simulink library "LIB_TF_G_12_StepControl"  (Simulink 8.6)
settings: Solver=ode45  StartTime=0.0  StopTime=10.0  RelTol=1e-3
PreLoadFcn:
  | if exist('tl_preloadfcn','file'), tl_preloadfcn(gcs,402); end
PostLoadFcn:
  | if exist('tl_postloadfcn','file'), tl_postloadfcn(gcs,402); end
undefined symbols (not defined in the file): ddv, u2, u3
libraries: tllib x4, LIB_TF_G_12_StepControl x1
(part 2 of 7)

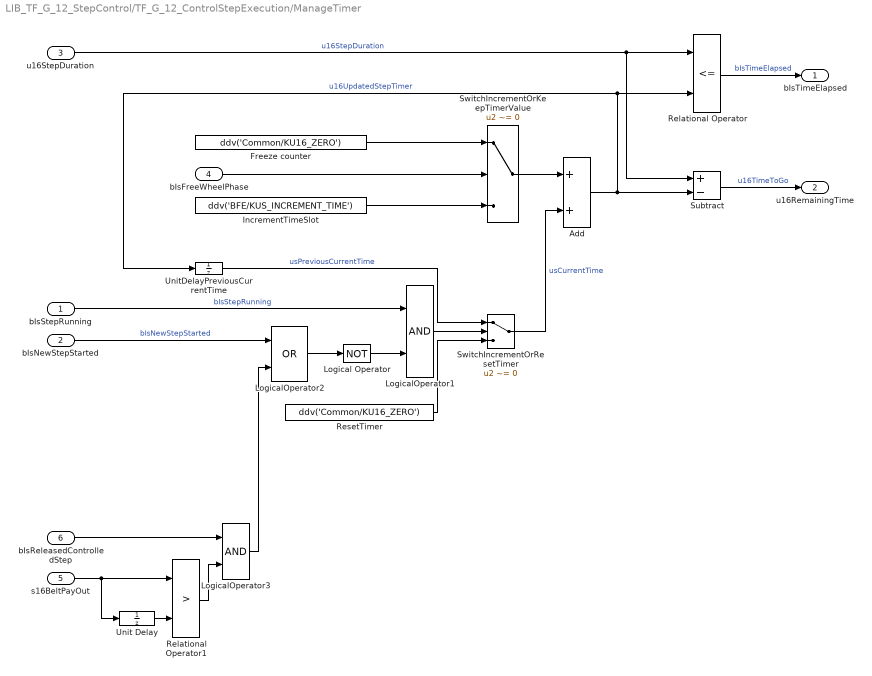
== system LIB_TF_G_12_StepControl/TF_G_12_ControlStepExecution/ManageTimer ==
  bIsStepRunning : Inport  RequirementInfo={} %GIDa_8099bea4_e8c1_4692_a6f9_d176147f505d
  bIsNewStepStarted : Inport  RequirementInfo={} %GIDa_5064309f_314f_43a7_8546_a3acea29a31d  Port=2
  u16StepDuration : Inport  RequirementInfo={} %GIDa_e2682689_4f53_4bd0_88ce_17de940b29c4  Port=3
  bIsFreeWheelPhase : Inport  RequirementInfo={} %GIDa_001aab12_c4fd_412a_b4f3_496d187da0da  Port=4
  s16BeltPayOut : Inport  RequirementInfo={} %GIDa_5cd29b0f_0f87_4eb9_b600_93c60318ecd2  Port=5  OutDataTypeStr=int16
  bIsReleasedControlledStep : Inport  RequirementInfo={} %GIDa_931de2e6_9d0e_47b7_b3af_677f90c0aa82  Port=6
  Add : Sum  RequirementInfo={} %GIDa_29793857_171b_4407_b062_784dd89fa0d8  OutDataTypeStr=uint16  SaturateOnIntegerOverflow=on  mask(TL_Sum){data={'output',{'name','u16UpdatedStepTimer','type','UInt16','checkmin',1,'checkmax',1},'autoscaling',{'mode',2},'date',735951.66800328705}}
      settings: AttributesFormatString=Saturation: %<SaturateOnIntegerOverflow>  CopyFcn=if exist('tl_reset_reviewflag','file')==2,tl_reset_reviewflag(gcbh);end  DeleteFcn=if exist('delete_tlblock','file')==2,delete_tlblock(gcbh);end  NameChangeFcn=if exist('rename_tlblock','file')==2,rename_tlblock(gcbh);end  OpenFcn=if exist('tl_open_blockdlg','file')==2,tl_open_blockdlg(gcbh);else,open_system(gcbh,'parameter');end
      mask Help: eval(['if exist(''tl_online_help'',''file'') == 2, tl_online_help(''Topic'',''TL_Sum''),else, web([''jar:file:///'',matlabroot,''/help/toolbox/simulink/help.jar!/slref/' lower(get_param(gcbh,'Blocktype')) '.html''], ''-helpbrowser''),end'])
      mask Display: plot([-0.05, 1.05, NaN, -0.05, 1.05],[.01, .01, NaN, .99, .99])
  Freeze counter : Constant  RequirementInfo={} %GIDa_b2dcc360_8c19_4b3e_bcea_e2e7e3051644  Value=ddv('Common/KU16_ZERO')  OutDataTypeStr=uint16  mask(TL_Constant){data={'output',{'variable','Common/KU16_ZERO'},'date',735951.66800163197}}
      settings: CopyFcn=if exist('tl_reset_reviewflag','file')==2,tl_reset_reviewflag(gcbh);end  DeleteFcn=if exist('delete_tlblock','file')==2,delete_tlblock(gcbh);end  NameChangeFcn=if exist('rename_tlblock','file')==2,rename_tlblock(gcbh);end  OpenFcn=if exist('tl_open_blockdlg','file')==2,tl_open_blockdlg(gcbh);else,open_system(gcbh,'parameter');end
      mask Help: eval(['if exist(''tl_online_help'',''file'') == 2, tl_online_help(''Topic'',''TL_Constant''),else, web([''jar:file:///'',matlabroot,''/help/toolbox/simulink/help.jar!/slref/' lower(get_param(gcbh,'Blocktype')) '.html''], ''-helpbrowser''),end'])
      mask Display: plot([-0.05, 1.05, NaN, -0.05, 1.05],[.01, .01, NaN, .99, .99])
  IncrementTimeSlot : Constant  RequirementInfo={} %GIDa_30227bc5_f72d_4077_9beb_be89df347bf6  Value=ddv('BFE/KUS_INCREMENT_TIME')  OutDataTypeStr=uint16  mask(TL_Constant){data={'output',{'variable','BFE/KUS_INCREMENT_TIME'},'date',735951.66800126154}}
      settings: CopyFcn=if exist('tl_reset_reviewflag','file')==2,tl_reset_reviewflag(gcbh);end  DeleteFcn=if exist('delete_tlblock','file')==2,delete_tlblock(gcbh);end  NameChangeFcn=if exist('rename_tlblock','file')==2,rename_tlblock(gcbh);end  OpenFcn=if exist('tl_open_blockdlg','file')==2,tl_open_blockdlg(gcbh);else,open_system(gcbh,'parameter');end
      mask Help: eval(['if exist(''tl_online_help'',''file'') == 2, tl_online_help(''Topic'',''TL_Constant''),else, web([''jar:file:///'',matlabroot,''/help/toolbox/simulink/help.jar!/slref/' lower(get_param(gcbh,'Blocktype')) '.html''], ''-helpbrowser''),end'])
      mask Display: plot([-0.05, 1.05, NaN, -0.05, 1.05],[.01, .01, NaN, .99, .99])
  Logical Operator : Logic  RequirementInfo={} %GIDa_a1686c55_b017_4ac8_bcb6_4b0a82067be0  Operator=NOT  Inputs=1  AllPortsSameDT=off  OutDataTypeStr=boolean  mask(TL_LogicalOperator){data={'date',735951.66800087958}}
      settings: DeleteFcn=if exist('delete_tlblock','file')==2,delete_tlblock(gcbh);end  NameChangeFcn=if exist('rename_tlblock','file')==2,rename_tlblock(gcbh);end  OpenFcn=if exist('tl_open_blockdlg','file')==2,tl_open_blockdlg(gcbh);else,open_system(gcbh,'parameter');end
      mask Help: eval(['if exist(''tl_online_help'',''file'') == 2, tl_online_help(''Topic'',''TL_LogicalOperator''),else, web([''jar:file:///'',matlabroot,''/help/toolbox/simulink/help.jar!/slref/' lower(get_param(gcbh,'Blocktype')) '.html''], ''-helpbrowser''),end'])
      mask Display: plot([-0.05, 1.05, NaN, -0.05, 1.05],[.01, .01, NaN, .99, .99])
  LogicalOperator1 : Logic  RequirementInfo={} %GIDa_4f8d19d4_46ad_40ac_a08b_006477df76af  AllPortsSameDT=off  OutDataTypeStr=boolean  mask(TL_LogicalOperator){data={'date',735951.66800062498}}
      settings: DeleteFcn=if exist('delete_tlblock','file')==2,delete_tlblock(gcbh);end  NameChangeFcn=if exist('rename_tlblock','file')==2,rename_tlblock(gcbh);end  OpenFcn=if exist('tl_open_blockdlg','file')==2,tl_open_blockdlg(gcbh);else,open_system(gcbh,'parameter');end
      mask Help: eval(['if exist(''tl_online_help'',''file'') == 2, tl_online_help(''Topic'',''TL_LogicalOperator''),else, web([''jar:file:///'',matlabroot,''/help/toolbox/simulink/help.jar!/slref/' lower(get_param(gcbh,'Blocktype')) '.html''], ''-helpbrowser''),end'])
      mask Display: plot([-0.05, 1.05, NaN, -0.05, 1.05],[.01, .01, NaN, .99, .99])
  LogicalOperator2 : Logic  RequirementInfo={} %GIDa_6e19c4e4_aaa7_45e7_9c6b_d801190fe024  Operator=OR  AllPortsSameDT=off  OutDataTypeStr=boolean  mask(TL_LogicalOperator){data={'date',735951.66800037038}}
      settings: DeleteFcn=if exist('delete_tlblock','file')==2,delete_tlblock(gcbh);end  NameChangeFcn=if exist('rename_tlblock','file')==2,rename_tlblock(gcbh);end  OpenFcn=if exist('tl_open_blockdlg','file')==2,tl_open_blockdlg(gcbh);else,open_system(gcbh,'parameter');end
      mask Help: eval(['if exist(''tl_online_help'',''file'') == 2, tl_online_help(''Topic'',''TL_LogicalOperator''),else, web([''jar:file:///'',matlabroot,''/help/toolbox/simulink/help.jar!/slref/' lower(get_param(gcbh,'Blocktype')) '.html''], ''-helpbrowser''),end'])
      mask Display: plot([-0.05, 1.05, NaN, -0.05, 1.05],[.01, .01, NaN, .99, .99])
  LogicalOperator3 : Logic  RequirementInfo={} %GIDa_591d57df_b6d7_4631_b542_675d73e86eef  AllPortsSameDT=off  OutDataTypeStr=boolean  mask(TL_LogicalOperator){data={'output',{'name','bIsConditionToRestartTimer'},'date',735951.66800011578}}
      settings: DeleteFcn=if exist('delete_tlblock','file')==2,delete_tlblock(gcbh);end  NameChangeFcn=if exist('rename_tlblock','file')==2,rename_tlblock(gcbh);end  OpenFcn=if exist('tl_open_blockdlg','file')==2,tl_open_blockdlg(gcbh);else,open_system(gcbh,'parameter');end
      mask Help: eval(['if exist(''tl_online_help'',''file'') == 2, tl_online_help(''Topic'',''TL_LogicalOperator''),else, web([''jar:file:///'',matlabroot,''/help/toolbox/simulink/help.jar!/slref/' lower(get_param(gcbh,'Blocktype')) '.html''], ''-helpbrowser''),end'])
      mask Display: plot([-0.05, 1.05, NaN, -0.05, 1.05],[.01, .01, NaN, .99, .99])
  Relational Operator : RelationalOperator  RequirementInfo={} %GIDa_885072fa_b492_4d65_aaa4_c1413b1c79d5  Operator=<=  OutDataTypeStr=boolean  mask(TL_RelationalOperator){data={'output',{'name','bIsTimerElapsed'},'date',735951.66799986106}}
      settings: DeleteFcn=if exist('delete_tlblock','file')==2,delete_tlblock(gcbh);end  NameChangeFcn=if exist('rename_tlblock','file')==2,rename_tlblock(gcbh);end  OpenFcn=if exist('tl_open_blockdlg','file')==2,tl_open_blockdlg(gcbh);else,open_system(gcbh,'parameter');end
      mask Help: eval(['if exist(''tl_online_help'',''file'') == 2, tl_online_help(''Topic'',''TL_RelationalOperator''),else, web([''jar:file:///'',matlabroot,''/help/toolbox/simulink/help.jar!/slref/' lower(get_param(gcbh,'Blocktype')) '.html''], ''-helpbrowser''),end'])
      mask Display: plot([-0.05, 1.05, NaN, -0.05, 1.05],[.01, .01, NaN, .99, .99])
  Relational Operator1 : RelationalOperator  RequirementInfo={} %GIDa_babd1620_4e70_45cd_94d3_ef9ded01dde4  Operator=>  OutDataTypeStr=boolean  mask(TL_RelationalOperator){data={'output',{'name','bBeltHasBeenPulled'},'date',735951.6679996181}}
      settings: DeleteFcn=if exist('delete_tlblock','file')==2,delete_tlblock(gcbh);end  NameChangeFcn=if exist('rename_tlblock','file')==2,rename_tlblock(gcbh);end  OpenFcn=if exist('tl_open_blockdlg','file')==2,tl_open_blockdlg(gcbh);else,open_system(gcbh,'parameter');end
      mask Help: eval(['if exist(''tl_online_help'',''file'') == 2, tl_online_help(''Topic'',''TL_RelationalOperator''),else, web([''jar:file:///'',matlabroot,''/help/toolbox/simulink/help.jar!/slref/' lower(get_param(gcbh,'Blocktype')) '.html''], ''-helpbrowser''),end'])
      mask Display: plot([-0.05, 1.05, NaN, -0.05, 1.05],[.01, .01, NaN, .99, .99])
  ResetTimer : Constant  RequirementInfo={} %GIDa_d400d14c_fedd_468a_9d55_b734797d539d  Value=ddv('Common/KU16_ZERO')  OutDataTypeStr=uint16  mask(TL_Constant){data={'output',{'variable','Common/KU16_ZERO'},'date',735951.66799936339}}
      settings: CopyFcn=if exist('tl_reset_reviewflag','file')==2,tl_reset_reviewflag(gcbh);end  DeleteFcn=if exist('delete_tlblock','file')==2,delete_tlblock(gcbh);end  NameChangeFcn=if exist('rename_tlblock','file')==2,rename_tlblock(gcbh);end  OpenFcn=if exist('tl_open_blockdlg','file')==2,tl_open_blockdlg(gcbh);else,open_system(gcbh,'parameter');end
      mask Help: eval(['if exist(''tl_online_help'',''file'') == 2, tl_online_help(''Topic'',''TL_Constant''),else, web([''jar:file:///'',matlabroot,''/help/toolbox/simulink/help.jar!/slref/' lower(get_param(gcbh,'Blocktype')) '.html''], ''-helpbrowser''),end'])
      mask Display: plot([-0.05, 1.05, NaN, -0.05, 1.05],[.01, .01, NaN, .99, .99])
  Subtract : Sum  RequirementInfo={} %GIDa_373c21ca_a1d9_4cd9_af23_8172f9ca01c1  Inputs=+-  OutDataTypeStr=uint16  SaturateOnIntegerOverflow=on  mask(TL_Sum){data={'output',{'name','u16RemainingTime','type','UInt16','checkmin',1,'checkmax',1},'autoscaling',{'mode',2},'date',735951.66799895838}}
      settings: CopyFcn=if exist('tl_reset_reviewflag','file')==2,tl_reset_reviewflag(gcbh);end  DeleteFcn=if exist('delete_tlblock','file')==2,delete_tlblock(gcbh);end  NameChangeFcn=if exist('rename_tlblock','file')==2,rename_tlblock(gcbh);end  OpenFcn=if exist('tl_open_blockdlg','file')==2,tl_open_blockdlg(gcbh);else,open_system(gcbh,'parameter');end
      mask Help: eval(['if exist(''tl_online_help'',''file'') == 2, tl_online_help(''Topic'',''TL_Sum''),else, web([''jar:file:///'',matlabroot,''/help/toolbox/simulink/help.jar!/slref/' lower(get_param(gcbh,'Blocktype')) '.html''], ''-helpbrowser''),end'])
      mask Display: plot([-0.05, 1.05, NaN, -0.05, 1.05],[.01, .01, NaN, .99, .99])
  SwitchIncrementOrKeepTimerValue : Switch  RequirementInfo={} %GIDa_30c2ac50_9b2c_44d9_a704_bb99cd63136e  Criteria=u2 ~= 0  OutDataTypeStr=uint16  SaturateOnIntegerOverflow=on  mask(TL_Switch){data={'output',{'name','u16TimerIncToApply','type','UInt16','checkmin',1,'checkmax',1},'autoscaling',{'mode',2},'date',735951.66799856478}}
      settings: CopyFcn=if exist('tl_reset_reviewflag','file')==2,tl_reset_reviewflag(gcbh);end  DeleteFcn=if exist('delete_tlblock','file')==2,delete_tlblock(gcbh);end  NameChangeFcn=if exist('rename_tlblock','file')==2,rename_tlblock(gcbh);end  OpenFcn=if exist('tl_open_blockdlg','file')==2,tl_open_blockdlg(gcbh);else,open_system(gcbh,'parameter');end
      mask Help: eval(['if exist(''tl_online_help'',''file'') == 2, tl_online_help(''Topic'',''TL_Switch''),else, web([''jar:file:///'',matlabroot,''/help/toolbox/simulink/help.jar!/slref/' lower(get_param(gcbh,'Blocktype')) '.html''], ''-helpbrowser''),end'])
      mask Display: plot([-0.05, 1.05, NaN, -0.05, 1.05],[.01, .01, NaN, .99, .99])
  SwitchIncrementOrResetTimer : Switch  RequirementInfo={} %GIDa_25344fa8_8921_4960_a2d3_faa64437b123  Criteria=u2 ~= 0  OutDataTypeStr=uint16  SaturateOnIntegerOverflow=on  mask(TL_Switch){data={'output',{'name','u16TimerOrigin','type','UInt16','checkmin',1,'checkmax',1},'autoscaling',{'mode',2},'date',735951.66799805558}}
      settings: CopyFcn=if exist('tl_reset_reviewflag','file')==2,tl_reset_reviewflag(gcbh);end  DeleteFcn=if exist('delete_tlblock','file')==2,delete_tlblock(gcbh);end  NameChangeFcn=if exist('rename_tlblock','file')==2,rename_tlblock(gcbh);end  OpenFcn=if exist('tl_open_blockdlg','file')==2,tl_open_blockdlg(gcbh);else,open_system(gcbh,'parameter');end
      mask Help: eval(['if exist(''tl_online_help'',''file'') == 2, tl_online_help(''Topic'',''TL_Switch''),else, web([''jar:file:///'',matlabroot,''/help/toolbox/simulink/help.jar!/slref/' lower(get_param(gcbh,'Blocktype')) '.html''], ''-helpbrowser''),end'])
      mask Display: plot([-0.05, 1.05, NaN, -0.05, 1.05],[.01, .01, NaN, .99, .99])
  Unit Delay : UnitDelay  RequirementInfo={} %GIDa_497777fa_c576_43da_9b3f_c02f48f7473a  SampleTime=-1  mask(TL_UnitDelay){data={'state',{'name','s16OldBeltPayOut'},'date',735951.66799752309}}
      settings: CopyFcn=if exist('tl_reset_reviewflag','file')==2,tl_reset_reviewflag(gcbh);end  DeleteFcn=if exist('delete_tlblock','file')==2,delete_tlblock(gcbh);end  NameChangeFcn=if exist('rename_tlblock','file')==2,rename_tlblock(gcbh);end  OpenFcn=if exist('tl_open_blockdlg','file')==2,tl_open_blockdlg(gcbh);else,open_system(gcbh,'parameter');end
      mask Help: eval(['if exist(''tl_online_help'',''file'') == 2, tl_online_help(''Topic'',''TL_UnitDelay''),else, web([''jar:file:///'',matlabroot,''/help/toolbox/simulink/help.jar!/slref/' lower(get_param(gcbh,'Blocktype')) '.html''], ''-helpbrowser''),end'])
      mask Display: plot([-0.05, 1.05, NaN, -0.05, 1.05],[.01, .01, NaN, .99, .99])
  UnitDelayPreviousCurrentTime : UnitDelay  RequirementInfo={} %GIDa_ddc782b0_2c14_4109_a1b3_6464a64ea15e  InitialCondition=ddv('Common/KU16_ZERO')  SampleTime=-1  mask(TL_UnitDelay){data={'output',{'type','UInt16'},'state',{'name','u16OldUpdatedStepTimer','type','UInt16'},'date',735951.6679969792}}
      settings: CopyFcn=if exist('tl_reset_reviewflag','file')==2,tl_reset_reviewflag(gcbh);end  DeleteFcn=if exist('delete_tlblock','file')==2,delete_tlblock(gcbh);end  NameChangeFcn=if exist('rename_tlblock','file')==2,rename_tlblock(gcbh);end  OpenFcn=if exist('tl_open_blockdlg','file')==2,tl_open_blockdlg(gcbh);else,open_system(gcbh,'parameter');end
      mask Help: eval(['if exist(''tl_online_help'',''file'') == 2, tl_online_help(''Topic'',''TL_UnitDelay''),else, web([''jar:file:///'',matlabroot,''/help/toolbox/simulink/help.jar!/slref/' lower(get_param(gcbh,'Blocktype')) '.html''], ''-helpbrowser''),end'])
      mask Display: plot([-0.05, 1.05, NaN, -0.05, 1.05],[.01, .01, NaN, .99, .99])
  bIsTimeElapsed : Outport  RequirementInfo={} %GIDa_70338377_5d6f_48f6_ad20_40eecd5f4ea6
  u16RemainingTime : Outport  RequirementInfo={} %GIDa_89bbad4f_06a6_4895_9511_fce3ce958955  Port=2
  wires:
  Subtract/1 -> u16RemainingTime/1  "u16TimeToGo"
  UnitDelayPreviousCurrentTime/1 -> SwitchIncrementOrResetTimer/1  "usPreviousCurrentTime"
  Freeze counter/1 -> SwitchIncrementOrKeepTimerValue/1
  IncrementTimeSlot/1 -> SwitchIncrementOrKeepTimerValue/3
  SwitchIncrementOrResetTimer/1 -> Add/2  "usCurrentTime"
  Add/1 -> Subtract/2, UnitDelayPreviousCurrentTime/1, Relational Operator/2  "u16UpdatedStepTimer"
  bIsFreeWheelPhase/1 -> SwitchIncrementOrKeepTimerValue/2
  SwitchIncrementOrKeepTimerValue/1 -> Add/1
  bIsNewStepStarted/1 -> LogicalOperator2/1  "bIsNewStepStarted"
  bIsStepRunning/1 -> LogicalOperator1/1  "bIsStepRunning"
  LogicalOperator1/1 -> SwitchIncrementOrResetTimer/2
  Relational Operator/1 -> bIsTimeElapsed/1  "bIsTimeElapsed"
  u16StepDuration/1 -> Subtract/1, Relational Operator/1  "u16StepDuration"
  ResetTimer/1 -> SwitchIncrementOrResetTimer/3
  LogicalOperator2/1 -> Logical Operator/1
  LogicalOperator3/1 -> LogicalOperator2/2
  bIsReleasedControlledStep/1 -> LogicalOperator3/1
  Relational Operator1/1 -> LogicalOperator3/2
  s16BeltPayOut/1 -> Relational Operator1/1, Unit Delay/1
  Unit Delay/1 -> Relational Operator1/2
  Logical Operator/1 -> LogicalOperator1/2

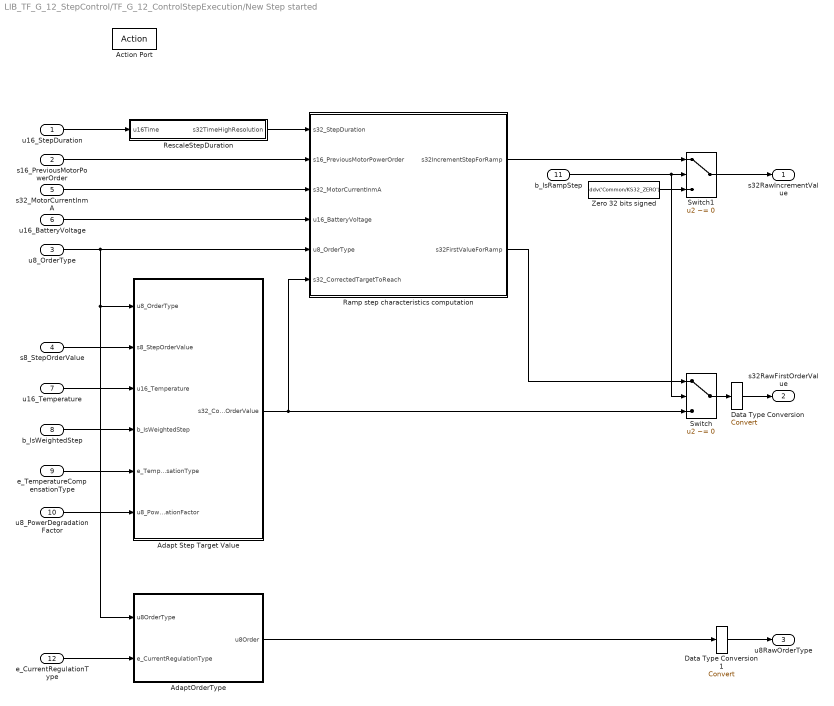
== system LIB_TF_G_12_StepControl/TF_G_12_ControlStepExecution/New Step started ==
  u16_StepDuration : Inport
  s16_PreviousMotorPowerOrder : Inport  Port=2
  u8_OrderType : Inport  Port=3
  s8_StepOrderValue : Inport  Port=4
  s32_MotorCurrentInmA : Inport  Port=5
  u16_BatteryVoltage : Inport  Port=6
  u16_Temperature : Inport  Port=7
  b_IsWeightedStep : Inport  Port=8
  e_TemperatureCompensationType : Inport  Port=9
  u8_PowerDegradationFactor : Inport  Port=10
  b_IsRampStep : Inport  Port=11
  e_CurrentRegulationType : Inport  Port=12
  Action Port : ActionPort
  Adapt Step Target Value : Subsystem  TreatAsAtomicUnit=on
  AdaptOrderType : Subsystem  RequirementInfo={} %GIDa_13dc65f5_0a95_4e88_a7b6_c4733fe3f649  TreatAsAtomicUnit=on
  Data Type Conversion : DataTypeConversion
  Data Type Conversion1 : DataTypeConversion
  Ramp step characteristics computation : Subsystem  TreatAsAtomicUnit=on
  RescaleStepDuration : Subsystem  RequirementInfo={} %GIDa_2ab98179_59e0_4a08_981b_442e90f39de3  TreatAsAtomicUnit=on
  Switch : Switch  Criteria=u2 ~= 0  OutDataTypeStr=int32  mask(TL_Switch){data={'output',{'type','Int32'},'date',735951.66796451388}}
      settings: CopyFcn=if exist('tl_reset_reviewflag','file')==2,tl_reset_reviewflag(gcbh);end  DeleteFcn=if exist('delete_tlblock','file')==2,delete_tlblock(gcbh);end  NameChangeFcn=if exist('rename_tlblock','file')==2,rename_tlblock(gcbh);end  OpenFcn=if exist('tl_open_blockdlg','file')==2,tl_open_blockdlg(gcbh);else,open_system(gcbh,'parameter');end
      mask Help: eval(['if exist(''tl_online_help'',''file'') == 2, tl_online_help(''Topic'',''TL_Switch''),else, web([''jar:file:///'',matlabroot,''/help/toolbox/simulink/help.jar!/slref/' lower(get_param(gcbh,'Blocktype')) '.html''], ''-helpbrowser''),end'])
      mask Display: plot([-0.05, 1.05, NaN, -0.05, 1.05],[.01, .01, NaN, .99, .99])
  Switch1 : Switch  Criteria=u2 ~= 0  mask(TL_Switch){data={'output',{'type','Int32'},'date',735951.66796400468}}
      settings: CopyFcn=if exist('tl_reset_reviewflag','file')==2,tl_reset_reviewflag(gcbh);end  DeleteFcn=if exist('delete_tlblock','file')==2,delete_tlblock(gcbh);end  NameChangeFcn=if exist('rename_tlblock','file')==2,rename_tlblock(gcbh);end  OpenFcn=if exist('tl_open_blockdlg','file')==2,tl_open_blockdlg(gcbh);else,open_system(gcbh,'parameter');end
      mask Help: eval(['if exist(''tl_online_help'',''file'') == 2, tl_online_help(''Topic'',''TL_Switch''),else, web([''jar:file:///'',matlabroot,''/help/toolbox/simulink/help.jar!/slref/' lower(get_param(gcbh,'Blocktype')) '.html''], ''-helpbrowser''),end'])
      mask Display: plot([-0.05, 1.05, NaN, -0.05, 1.05],[.01, .01, NaN, .99, .99])
  Zero 32 bits signed : Constant  Value=ddv('Common/KS32_ZERO')  mask(TL_Constant){data={'output',{'variable','Common/KS32_ZERO'},'date',735951.66796349536}}
      settings: CopyFcn=if exist('tl_reset_reviewflag','file')==2,tl_reset_reviewflag(gcbh);end  DeleteFcn=if exist('delete_tlblock','file')==2,delete_tlblock(gcbh);end  NameChangeFcn=if exist('rename_tlblock','file')==2,rename_tlblock(gcbh);end  OpenFcn=if exist('tl_open_blockdlg','file')==2,tl_open_blockdlg(gcbh);else,open_system(gcbh,'parameter');end
      mask Help: eval(['if exist(''tl_online_help'',''file'') == 2, tl_online_help(''Topic'',''TL_Constant''),else, web([''jar:file:///'',matlabroot,''/help/toolbox/simulink/help.jar!/slref/' lower(get_param(gcbh,'Blocktype')) '.html''], ''-helpbrowser''),end'])
      mask Display: plot([-0.05, 1.05, NaN, -0.05, 1.05],[.01, .01, NaN, .99, .99])
  s32RawIncrementValue : Outport  InitialOutput=0
  s32RawFirstOrderValue : Outport  Port=2  InitialOutput=0
  u8RawOrderType : Outport  Port=3  InitialOutput=0
  wires:
  Data Type Conversion1/1 -> u8RawOrderType/1
  AdaptOrderType/1(u8Order) -> Data Type Conversion1/1
  u8_OrderType/1 -> AdaptOrderType/1(u8OrderType), Adapt Step Target Value/1(u8_OrderType), Ramp step characteristics computation/5(u8_OrderType)
  s8_StepOrderValue/1 -> Adapt Step Target Value/2(s8_StepOrderValue)
  u16_Temperature/1 -> Adapt Step Target Value/3(u16_Temperature)
  b_IsWeightedStep/1 -> Adapt Step Target Value/4(b_IsWeightedStep)
  e_TemperatureCompensationType/1 -> Adapt Step Target Value/5(e_TemperatureCompensationType)
  u8_PowerDegradationFactor/1 -> Adapt Step Target Value/6(u8_PowerDegradationFactor)
  u16_StepDuration/1 -> RescaleStepDuration/1(u16Time)
  Switch1/1 -> s32RawIncrementValue/1
  Switch/1 -> Data Type Conversion/1
  b_IsRampStep/1 -> Switch1/2, Switch/2
  Adapt Step Target Value/1(s32_CorrectedOrderValue) -> Switch/3, Ramp step characteristics computation/6(s32_CorrectedTargetToReach)
  Zero 32 bits signed/1 -> Switch1/3
  Ramp step characteristics computation/1(s32IncrementStepForRamp) -> Switch1/1
  Ramp step characteristics computation/2(s32FirstValueForRamp) -> Switch/1
  s16_PreviousMotorPowerOrder/1 -> Ramp step characteristics computation/2(s16_PreviousMotorPowerOrder)
  RescaleStepDuration/1(s32TimeHighResolution) -> Ramp step characteristics computation/1(s32_StepDuration)
  u16_BatteryVoltage/1 -> Ramp step characteristics computation/4(u16_BatteryVoltage)
  s32_MotorCurrentInmA/1 -> Ramp step characteristics computation/3(s32_MotorCurrentInmA)
  e_CurrentRegulationType/1 -> AdaptOrderType/2(e_CurrentRegulationType)
  Data Type Conversion/1 -> s32RawFirstOrderValue/1

== system LIB_TF_G_12_StepControl/TF_G_12_ControlStepExecution/No step executed ==
  Action Port : ActionPort
  Motor power order shall be reset : Constant  Value=ddv('Common/KS32_ZERO')  mask(TL_Constant){data={'output',{'variable','Common/KS32_ZERO'},'date',735951.66796312504}}
      settings: CopyFcn=if exist('tl_reset_reviewflag','file')==2,tl_reset_reviewflag(gcbh);end  DeleteFcn=if exist('delete_tlblock','file')==2,delete_tlblock(gcbh);end  NameChangeFcn=if exist('rename_tlblock','file')==2,rename_tlblock(gcbh);end  OpenFcn=if exist('tl_open_blockdlg','file')==2,tl_open_blockdlg(gcbh);else,open_system(gcbh,'parameter');end
      mask Help: eval(['if exist(''tl_online_help'',''file'') == 2, tl_online_help(''Topic'',''TL_Constant''),else, web([''jar:file:///'',matlabroot,''/help/toolbox/simulink/help.jar!/slref/' lower(get_param(gcbh,'Blocktype')) '.html''], ''-helpbrowser''),end'])
      mask Display: plot([-0.05, 1.05, NaN, -0.05, 1.05],[.01, .01, NaN, .99, .99])
  Motor power order shall be reset1 : Constant  Value=ddv('Common/KS32_ZERO')  mask(TL_Constant){data={'output',{'variable','Common/KS32_ZERO'},'date',735951.66796274309}}
      settings: CopyFcn=if exist('tl_reset_reviewflag','file')==2,tl_reset_reviewflag(gcbh);end  DeleteFcn=if exist('delete_tlblock','file')==2,delete_tlblock(gcbh);end  NameChangeFcn=if exist('rename_tlblock','file')==2,rename_tlblock(gcbh);end  OpenFcn=if exist('tl_open_blockdlg','file')==2,tl_open_blockdlg(gcbh);else,open_system(gcbh,'parameter');end
      mask Help: eval(['if exist(''tl_online_help'',''file'') == 2, tl_online_help(''Topic'',''TL_Constant''),else, web([''jar:file:///'',matlabroot,''/help/toolbox/simulink/help.jar!/slref/' lower(get_param(gcbh,'Blocktype')) '.html''], ''-helpbrowser''),end'])
      mask Display: plot([-0.05, 1.05, NaN, -0.05, 1.05],[.01, .01, NaN, .99, .99])
  No step Order Type : Constant  Value=ddv('BFE/Step_Def/KU8_NO_STEP_TYPE')  OutDataTypeStr=uint8  mask(TL_Constant){data={'output',{'variable','BFE/Step_Def/KU8_NO_STEP_TYPE'},'date',735951.66796237265}}
      settings: CopyFcn=if exist('tl_reset_reviewflag','file')==2,tl_reset_reviewflag(gcbh);end  DeleteFcn=if exist('delete_tlblock','file')==2,delete_tlblock(gcbh);end  NameChangeFcn=if exist('rename_tlblock','file')==2,rename_tlblock(gcbh);end  OpenFcn=if exist('tl_open_blockdlg','file')==2,tl_open_blockdlg(gcbh);else,open_system(gcbh,'parameter');end
      mask Help: eval(['if exist(''tl_online_help'',''file'') == 2, tl_online_help(''Topic'',''TL_Constant''),else, web([''jar:file:///'',matlabroot,''/help/toolbox/simulink/help.jar!/slref/' lower(get_param(gcbh,'Blocktype')) '.html''], ''-helpbrowser''),end'])
      mask Display: plot([-0.05, 1.05, NaN, -0.05, 1.05],[.01, .01, NaN, .99, .99])
  s32RawIncrementValue : Outport  InitialOutput=0
  s32RawFirstOrderValue : Outport  Port=2  InitialOutput=0
  u8RawOrderType : Outport  Port=3  InitialOutput=0
  wires:
  No step Order Type/1 -> u8RawOrderType/1
  Motor power order shall be reset/1 -> s32RawIncrementValue/1
  Motor power order shall be reset1/1 -> s32RawFirstOrderValue/1

== system LIB_TF_G_12_StepControl/TF_G_12_ControlStepExecution/Step execution continues ==
  s32PrevRawIncrementValue : Inport
  s32PrevRawFirstOrderValue : Inport  Port=2
  u8PrevRawOrderType : Inport  Port=3
  Action Port : ActionPort
  s32RawIncrementValue : Outport  InitialOutput=0
  s32RawFirstOrderValue : Outport  Port=2  InitialOutput=0
  u8RawOrderType : Outport  Port=3  InitialOutput=0
  wires:
  u8PrevRawOrderType/1 -> u8RawOrderType/1
  s32PrevRawIncrementValue/1 -> s32RawIncrementValue/1
  s32PrevRawFirstOrderValue/1 -> s32RawFirstOrderValue/1

== system LIB_TF_G_12_StepControl/TF_G_12_ManageEndingStep/No step running ==
  Action Port : ActionPort  RequirementInfo={} %GIDa_c65bb53b_804b_41d1_b52e_bea7bc0c5513
  KB_TRUE : Constant  RequirementInfo={} %GIDa_6933dfa3_0ae3_4e05_b095_5f75714e2f16  Value=ddv('BFE/KB_TRUE')  OutDataTypeStr=boolean  mask(TL_Constant){data={'output',{'variable','BFE/KB_TRUE'},'date',735951.66848581017}}
      settings: CopyFcn=if exist('tl_reset_reviewflag','file')==2,tl_reset_reviewflag(gcbh);end  DeleteFcn=if exist('delete_tlblock','file')==2,delete_tlblock(gcbh);end  NameChangeFcn=if exist('rename_tlblock','file')==2,rename_tlblock(gcbh);end  OpenFcn=if exist('tl_open_blockdlg','file')==2,tl_open_blockdlg(gcbh);else,open_system(gcbh,'parameter');end
      mask Help: eval(['if exist(''tl_online_help'',''file'') == 2, tl_online_help(''Topic'',''TL_Constant''),else, web([''jar:file:///'',matlabroot,''/help/toolbox/simulink/help.jar!/slref/' lower(get_param(gcbh,'Blocktype')) '.html''], ''-helpbrowser''),end'])
      mask Display: plot([-0.05, 1.05, NaN, -0.05, 1.05],[.01, .01, NaN, .99, .99])
  bInterruptStep : Outport  RequirementInfo={} %GIDa_2df0479f_740e_423b_b079_8b181e076bef  InitialOutput=1
  wires:
  KB_TRUE/1 -> bInterruptStep/1

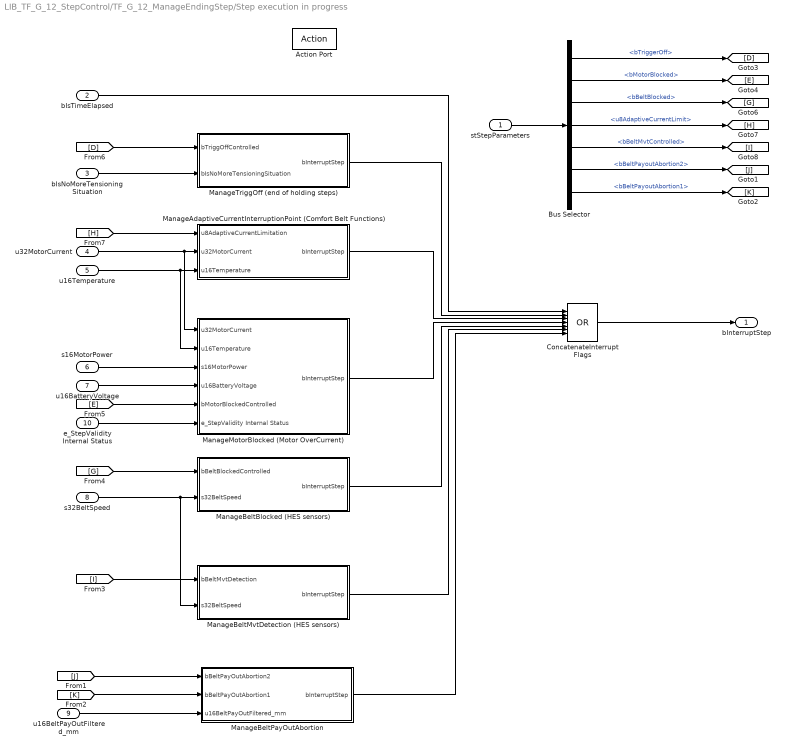
== system LIB_TF_G_12_StepControl/TF_G_12_ManageEndingStep/Step execution in progress ==
  stStepParameters : Inport  RequirementInfo={} %GIDa_bee7fcd0_5576_40d4_b001_007e9b2676d5
  bIsTimeElapsed : Inport  RequirementInfo={} %GIDa_c850359e_5352_4d8f_8c8a_0570fbf850c3  Port=2
  bIsNoMoreTensioningSituation : Inport  RequirementInfo={} %GIDa_22d072f3_e6ca_40a8_9550_a3f21e6ba458  Port=3
  u32MotorCurrent : Inport  RequirementInfo={} %GIDa_ae72be22_6924_4b19_8898_d7dbc6aa64b9  Port=4
  u16Temperature : Inport  RequirementInfo={} %GIDa_ef219c60_beb7_4c0f_8d72_df139f88d559  Port=5
  s16MotorPower : Inport  RequirementInfo={} %GIDa_b3306dfd_64f7_49f6_9ab4_e7bad97fcf30  Port=6
  u16BatteryVoltage : Inport  RequirementInfo={} %GIDa_133bcd52_a802_46c5_8b03_ce9e3adf493b  Port=7
  s32BeltSpeed : Inport  RequirementInfo={} %GIDa_e56246d3_8198_499b_88d1_aef53e6ce9c0  Port=8
  u16BeltPayOutFiltered_mm : Inport  RequirementInfo={} %GIDa_e28dd7cf_b0d0_426a_b3ae_bcdc9eda29f0  Port=9
  e_StepValidity Internal Status : Inport  RequirementInfo={} %GIDa_ec48f654_3f2a_47e8_a03b_effd5e2f0ea1  Port=10
  Action Port : ActionPort  RequirementInfo={} %GIDa_363ed3e8_01c7_48bc_abe5_8b37d647626f
  Bus Selector : BusSelector  RequirementInfo={} %GIDa_50b9a37a_e534_4f27_a694_a44dbdb5cd10  OutputSignals=bTriggerOff,bMotorBlocked,bBeltBlocked,u8AdaptiveCurrentLimit,bBeltMvtControlled,bBeltPayoutAbortion2,bBeltPayoutAbortion1
  ConcatenateInterruptFlags : Logic  RequirementInfo={} %GIDa_27383bb1_6cf6_4314_9ee5_d7eb641c5f76  Operator=OR  Inputs=7  AllPortsSameDT=off  OutDataTypeStr=boolean  mask(TL_LogicalOperator){data={'date',735951.66848458338}}
      settings: DeleteFcn=if exist('delete_tlblock','file')==2,delete_tlblock(gcbh);end  NameChangeFcn=if exist('rename_tlblock','file')==2,rename_tlblock(gcbh);end  OpenFcn=if exist('tl_open_blockdlg','file')==2,tl_open_blockdlg(gcbh);else,open_system(gcbh,'parameter');end
      mask Help: eval(['if exist(''tl_online_help'',''file'') == 2, tl_online_help(''Topic'',''TL_LogicalOperator''),else, web([''jar:file:///'',matlabroot,''/help/toolbox/simulink/help.jar!/slref/' lower(get_param(gcbh,'Blocktype')) '.html''], ''-helpbrowser''),end'])
      mask Display: plot([-0.05, 1.05, NaN, -0.05, 1.05],[.01, .01, NaN, .99, .99])
  ManageAdaptiveCurrentInterruptionPoint (Comfort Belt Functions) : Subsystem  RequirementInfo={} %GIDa_1cd97ecc_1cbf_46a6_a637_a3857b006779  TreatAsAtomicUnit=on
  ManageBeltBlocked (HES sensors) : Subsystem  RequirementInfo={} %GIDa_3b53e2f4_db0e_4732_bb83_ba2e5dae0770  TreatAsAtomicUnit=on
  ManageBeltMvtDetection (HES sensors) : Subsystem  RequirementInfo={} %GIDa_15e6ce68_08e2_44b6_bc8d_dd9e3b170fcc  TreatAsAtomicUnit=on
  ManageBeltPayOutAbortion : Subsystem  RequirementInfo={} %GIDa_a09f03a1_6db1_492c_8b3a_841a7e106edb  TreatAsAtomicUnit=on
  ManageMotorBlocked (Motor OverCurrent) : Subsystem  RequirementInfo={} %GIDa_5a169fa5_3576_4d28_a05d_a55595eeddc0  TreatAsAtomicUnit=on
  ManageTriggOff (end of holding steps) : Subsystem  RequirementInfo={} %GIDa_dd093c88_4480_4878_aadb_96f2b4aa36fe  TreatAsAtomicUnit=on
  bInterruptStep : Outport  RequirementInfo={} %GIDa_beb40c9e_ceaf_4736_be8f_4d5ae61f6c32
  wires:
  ConcatenateInterruptFlags/1 -> bInterruptStep/1
  bIsTimeElapsed/1 -> ConcatenateInterruptFlags/1
  Bus Selector/1 -> [D]  "<bTriggerOff>"
  Bus Selector/2 -> [E]  "<bMotorBlocked>"
  Bus Selector/3 -> [G]  "<bBeltBlocked>"
  Bus Selector/4 -> [H]  "<u8AdaptiveCurrentLimit>"
  Bus Selector/5 -> [I]  "<bBeltMvtControlled>"
  stStepParameters/1 -> Bus Selector/1
  [D] -> ManageTriggOff (end of holding steps)/1(bTriggOffControlled)
  bIsNoMoreTensioningSituation/1 -> ManageTriggOff (end of holding steps)/2(bIsNoMoreTensioningSituation)
  ManageTriggOff (end of holding steps)/1(bInterruptStep) -> ConcatenateInterruptFlags/2
  [H] -> ManageAdaptiveCurrentInterruptionPoint (Comfort Belt Functions)/1(u8AdaptiveCurrentLimitation)
  ManageAdaptiveCurrentInterruptionPoint (Comfort Belt Functions)/1(bInterruptStep) -> ConcatenateInterruptFlags/3
  u32MotorCurrent/1 -> ManageAdaptiveCurrentInterruptionPoint (Comfort Belt Functions)/2(u32MotorCurrent), ManageMotorBlocked (Motor OverCurrent)/1(u32MotorCurrent)
  u16Temperature/1 -> ManageAdaptiveCurrentInterruptionPoint (Comfort Belt Functions)/3(u16Temperature), ManageMotorBlocked (Motor OverCurrent)/2(u16Temperature)
  [G] -> ManageBeltBlocked (HES sensors)/1(bBeltBlockedControlled)
  s32BeltSpeed/1 -> ManageBeltBlocked (HES sensors)/2(s32BeltSpeed), ManageBeltMvtDetection (HES sensors)/2(s32BeltSpeed)
  [I] -> ManageBeltMvtDetection (HES sensors)/1(bBeltMvtDetection)
  [E] -> ManageMotorBlocked (Motor OverCurrent)/5(bMotorBlockedControlled)
  u16BatteryVoltage/1 -> ManageMotorBlocked (Motor OverCurrent)/4(u16BatteryVoltage)
  s16MotorPower/1 -> ManageMotorBlocked (Motor OverCurrent)/3(s16MotorPower)
  ManageMotorBlocked (Motor OverCurrent)/1(bInterruptStep) -> ConcatenateInterruptFlags/4
  ManageBeltBlocked (HES sensors)/1(bInterruptStep) -> ConcatenateInterruptFlags/5
  ManageBeltMvtDetection (HES sensors)/1(bInterruptStep) -> ConcatenateInterruptFlags/6
  u16BeltPayOutFiltered_mm/1 -> ManageBeltPayOutAbortion/3(u16BeltPayOutFiltered_mm)
  [J] -> ManageBeltPayOutAbortion/1(bBeltPayOutAbortion2)
  [K] -> ManageBeltPayOutAbortion/2(bBeltPayOutAbortion1)
  ManageBeltPayOutAbortion/1(bInterruptStep) -> ConcatenateInterruptFlags/7
  Bus Selector/6 -> [J]  "<bBeltPayoutAbortion2>"
  Bus Selector/7 -> [K]  "<bBeltPayoutAbortion1>"
  e_StepValidity Internal Status/1 -> ManageMotorBlocked (Motor OverCurrent)/6(e_StepValidity Internal Status)

== system LIB_TF_G_12_StepControl/TF_G_12_ControlStepExecution/Extrapolate Next Consign/SubsystemDetectConsignsChange ==
  lFirstOrder : Inport  RequirementInfo={} %GIDa_c6d97c01_3bec_4185_96f0_675475ba74ca
  lIncrement : Inport  RequirementInfo={} %GIDa_84debdd4_711e_453d_afc6_e0217592a3f0  Port=2
  Logical Operator : Logic  RequirementInfo={} %GIDa_6ecfbbbb_12c2_482c_84a5_12b01e601fd0  Operator=OR  AllPortsSameDT=off  OutDataTypeStr=boolean  mask(TL_LogicalOperator){data={'output',{'name','bNewConsigns'},'date',735951.66800856485}}
      settings: DeleteFcn=if exist('delete_tlblock','file')==2,delete_tlblock(gcbh);end  NameChangeFcn=if exist('rename_tlblock','file')==2,rename_tlblock(gcbh);end  OpenFcn=if exist('tl_open_blockdlg','file')==2,tl_open_blockdlg(gcbh);else,open_system(gcbh,'parameter');end
      mask Help: eval(['if exist(''tl_online_help'',''file'') == 2, tl_online_help(''Topic'',''TL_LogicalOperator''),else, web([''jar:file:///'',matlabroot,''/help/toolbox/simulink/help.jar!/slref/' lower(get_param(gcbh,'Blocktype')) '.html''], ''-helpbrowser''),end'])
      mask Display: plot([-0.05, 1.05, NaN, -0.05, 1.05],[.01, .01, NaN, .99, .99])
  Relational Operator : RelationalOperator  RequirementInfo={} %GIDa_d51074f0_92a9_4b3d_850c_6ad92c1829e8  Operator=~=  OutDataTypeStr=boolean  mask(TL_RelationalOperator){data={'date',735951.66800831014}}
      settings: DeleteFcn=if exist('delete_tlblock','file')==2,delete_tlblock(gcbh);end  NameChangeFcn=if exist('rename_tlblock','file')==2,rename_tlblock(gcbh);end  OpenFcn=if exist('tl_open_blockdlg','file')==2,tl_open_blockdlg(gcbh);else,open_system(gcbh,'parameter');end
      mask Help: eval(['if exist(''tl_online_help'',''file'') == 2, tl_online_help(''Topic'',''TL_RelationalOperator''),else, web([''jar:file:///'',matlabroot,''/help/toolbox/simulink/help.jar!/slref/' lower(get_param(gcbh,'Blocktype')) '.html''], ''-helpbrowser''),end'])
      mask Display: plot([-0.05, 1.05, NaN, -0.05, 1.05],[.01, .01, NaN, .99, .99])
  Relational Operator1 : RelationalOperator  RequirementInfo={} %GIDa_5926b92f_b4c2_4445_8751_5a0ddf4b4fde  Operator=~=  OutDataTypeStr=boolean  mask(TL_RelationalOperator){data={'date',735951.66800806718}}
      settings: DeleteFcn=if exist('delete_tlblock','file')==2,delete_tlblock(gcbh);end  NameChangeFcn=if exist('rename_tlblock','file')==2,rename_tlblock(gcbh);end  OpenFcn=if exist('tl_open_blockdlg','file')==2,tl_open_blockdlg(gcbh);else,open_system(gcbh,'parameter');end
      mask Help: eval(['if exist(''tl_online_help'',''file'') == 2, tl_online_help(''Topic'',''TL_RelationalOperator''),else, web([''jar:file:///'',matlabroot,''/help/toolbox/simulink/help.jar!/slref/' lower(get_param(gcbh,'Blocktype')) '.html''], ''-helpbrowser''),end'])
      mask Display: plot([-0.05, 1.05, NaN, -0.05, 1.05],[.01, .01, NaN, .99, .99])
  Unit Delay : UnitDelay  RequirementInfo={} %GIDa_ce67a684_7292_43d1_b9e2_ddcc1d40e5e2  SampleTime=-1  mask(TL_UnitDelay){data={'output',{'type','Int32'},'state',{'name','s32OldIncrement','type','Int32'},'date',735951.66800777777}}
      settings: CopyFcn=if exist('tl_reset_reviewflag','file')==2,tl_reset_reviewflag(gcbh);end  DeleteFcn=if exist('delete_tlblock','file')==2,delete_tlblock(gcbh);end  NameChangeFcn=if exist('rename_tlblock','file')==2,rename_tlblock(gcbh);end  OpenFcn=if exist('tl_open_blockdlg','file')==2,tl_open_blockdlg(gcbh);else,open_system(gcbh,'parameter');end
      mask Help: eval(['if exist(''tl_online_help'',''file'') == 2, tl_online_help(''Topic'',''TL_UnitDelay''),else, web([''jar:file:///'',matlabroot,''/help/toolbox/simulink/help.jar!/slref/' lower(get_param(gcbh,'Blocktype')) '.html''], ''-helpbrowser''),end'])
      mask Display: plot([-0.05, 1.05, NaN, -0.05, 1.05],[.01, .01, NaN, .99, .99])
  Unit Delay1 : UnitDelay  RequirementInfo={} %GIDa_a69bd70f_c50d_4d42_907d_ff8511c10c46  SampleTime=-1  mask(TL_UnitDelay){data={'output',{'type','Int32'},'state',{'name','s32OldFirstOrder','type','Int32'},'date',735951.6680072454}}
      settings: CopyFcn=if exist('tl_reset_reviewflag','file')==2,tl_reset_reviewflag(gcbh);end  DeleteFcn=if exist('delete_tlblock','file')==2,delete_tlblock(gcbh);end  NameChangeFcn=if exist('rename_tlblock','file')==2,rename_tlblock(gcbh);end  OpenFcn=if exist('tl_open_blockdlg','file')==2,tl_open_blockdlg(gcbh);else,open_system(gcbh,'parameter');end
      mask Help: eval(['if exist(''tl_online_help'',''file'') == 2, tl_online_help(''Topic'',''TL_UnitDelay''),else, web([''jar:file:///'',matlabroot,''/help/toolbox/simulink/help.jar!/slref/' lower(get_param(gcbh,'Blocktype')) '.html''], ''-helpbrowser''),end'])
      mask Display: plot([-0.05, 1.05, NaN, -0.05, 1.05],[.01, .01, NaN, .99, .99])
  bAreConsignsChanged : Outport  RequirementInfo={} %GIDa_744b5259_caed_4eb9_99b0_ba8ed55267b5
  wires:
  lFirstOrder/1 -> Relational Operator1/1, Unit Delay1/1
  lIncrement/1 -> Relational Operator/1, Unit Delay/1
  Unit Delay/1 -> Relational Operator/2
  Unit Delay1/1 -> Relational Operator1/2
  Logical Operator/1 -> bAreConsignsChanged/1
  Relational Operator/1 -> Logical Operator/1
  Relational Operator1/1 -> Logical Operator/2

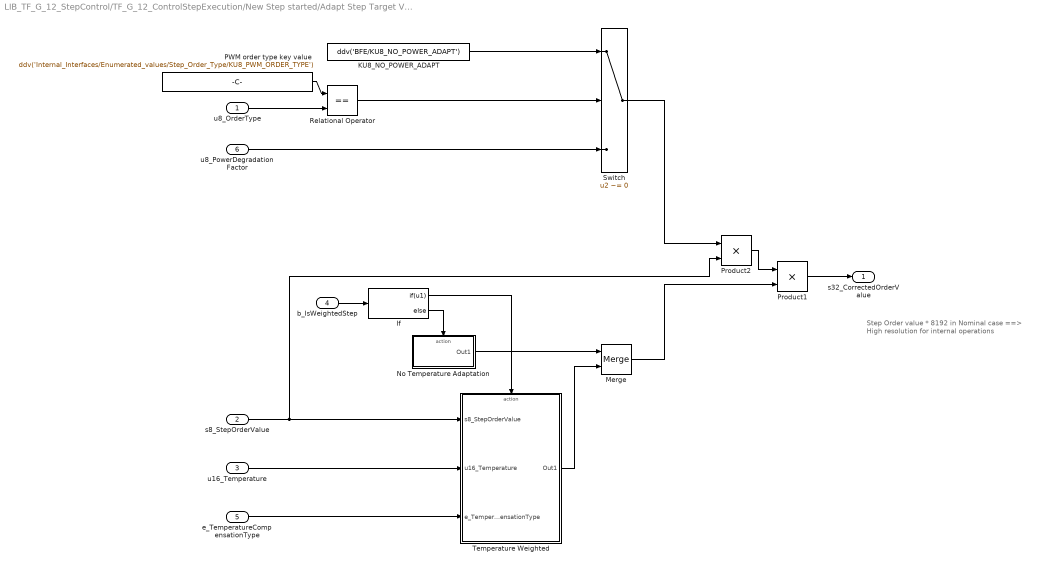
== system LIB_TF_G_12_StepControl/TF_G_12_ControlStepExecution/New Step started/Adapt Step Target Value ==
  note: Step Order value * 8192 in Nominal case
      | ==> High resolution for internal operations
  u8_OrderType : Inport
  s8_StepOrderValue : Inport  Port=2
  u16_Temperature : Inport  Port=3
  b_IsWeightedStep : Inport  Port=4
  e_TemperatureCompensationType : Inport  Port=5
  u8_PowerDegradationFactor : Inport  Port=6
  If : If  IfExpression=u1
  KU8_NO_POWER_ADAPT : Constant  RequirementInfo={} %GIDa_2b2c29ee_3c7c_443f_bc3d_925541208a4b  Value=ddv('BFE/KU8_NO_POWER_ADAPT')  OutDataTypeStr=uint8  mask(TL_Constant){data={'output',{'variable','BFE/KU8_NO_POWER_ADAPT'},'date',735951.66799531248}}
      settings: CopyFcn=if exist('tl_reset_reviewflag','file')==2,tl_reset_reviewflag(gcbh);end  DeleteFcn=if exist('delete_tlblock','file')==2,delete_tlblock(gcbh);end  NameChangeFcn=if exist('rename_tlblock','file')==2,rename_tlblock(gcbh);end  OpenFcn=if exist('tl_open_blockdlg','file')==2,tl_open_blockdlg(gcbh);else,open_system(gcbh,'parameter');end
      mask Help: eval(['if exist(''tl_online_help'',''file'') == 2, tl_online_help(''Topic'',''TL_Constant''),else, web([''jar:file:///'',matlabroot,''/help/toolbox/simulink/help.jar!/slref/' lower(get_param(gcbh,'Blocktype')) '.html''], ''-helpbrowser''),end'])
      mask Display: plot([-0.05, 1.05, NaN, -0.05, 1.05],[.01, .01, NaN, .99, .99])
  Merge : Merge  InitialOutput=64  mask(TL_Merge){data={'output',{'name','u8TemperatureCorrectionFactor'},'date',735951.66799490736}}
      settings: CopyFcn=if exist('tl_reset_reviewflag','file')==2,tl_reset_reviewflag(gcbh);end  DeleteFcn=if exist('delete_tlblock','file')==2,delete_tlblock(gcbh);end  NameChangeFcn=if exist('rename_tlblock','file')==2,rename_tlblock(gcbh);end  OpenFcn=if exist('tl_open_blockdlg','file')==2,tl_open_blockdlg(gcbh);else,open_system(gcbh,'parameter');end
      mask Help: eval(['if exist(''tl_online_help'',''file'') == 2, tl_online_help(''Topic'',''TL_Merge''),else, web([''jar:file:///'',matlabroot,''/help/toolbox/simulink/help.jar!/slref/' lower(get_param(gcbh,'Blocktype')) '.html''], ''-helpbrowser''),end'])
      mask Display: plot([-0.05, 1.05, NaN, -0.05, 1.05],[.01, .01, NaN, .99, .99])
  No Temperature Adaptation : Subsystem  TreatAsAtomicUnit=on
  PWM order type key value : Constant  Value=ddv('Internal_Interfaces/Enumerated_values/Step_Order_Type/KU8_PWM_ORDER_TYPE')  mask(TL_Constant){data={'output',{'variable','Internal_Interfaces/Enumerated_values/Step_Order_Type/KU8_PWM_ORDER_TYPE'},'date',735951.66799416672}}
      settings: CopyFcn=if exist('tl_reset_reviewflag','file')==2,tl_reset_reviewflag(gcbh);end  DeleteFcn=if exist('delete_tlblock','file')==2,delete_tlblock(gcbh);end  NameChangeFcn=if exist('rename_tlblock','file')==2,rename_tlblock(gcbh);end  OpenFcn=if exist('tl_open_blockdlg','file')==2,tl_open_blockdlg(gcbh);else,open_system(gcbh,'parameter');end
      mask Help: eval(['if exist(''tl_online_help'',''file'') == 2, tl_online_help(''Topic'',''TL_Constant''),else, web([''jar:file:///'',matlabroot,''/help/toolbox/simulink/help.jar!/slref/' lower(get_param(gcbh,'Blocktype')) '.html''], ''-helpbrowser''),end'])
      mask Display: plot([-0.05, 1.05, NaN, -0.05, 1.05],[.01, .01, NaN, .99, .99])
  Product1 : Product  Inputs=**  RndMeth=Zero  mask(TL_Product){data={'output',{'name','s32CorrectedStepOrderValue','type','Int32'},'date',735951.66799377312}}
      settings: CopyFcn=if exist('tl_reset_reviewflag','file')==2,tl_reset_reviewflag(gcbh);end  DeleteFcn=if exist('delete_tlblock','file')==2,delete_tlblock(gcbh);end  NameChangeFcn=if exist('rename_tlblock','file')==2,rename_tlblock(gcbh);end  OpenFcn=if exist('tl_open_blockdlg','file')==2,tl_open_blockdlg(gcbh);else,open_system(gcbh,'parameter');end
      mask Help: eval(['if exist(''tl_online_help'',''file'') == 2, tl_online_help(''Topic'',''TL_Product''),else, web([''jar:file:///'',matlabroot,''/help/toolbox/simulink/help.jar!/slref/' lower(get_param(gcbh,'Blocktype')) '.html''], ''-helpbrowser''),end'])
      mask Display: plot([-0.05, 1.05, NaN, -0.05, 1.05],[.01, .01, NaN, .99, .99])
  Product2 : Product  Inputs=**  RndMeth=Zero  mask(TL_Product){data={'output',{'type','Int32'},'date',735951.66799340281}}
      settings: CopyFcn=if exist('tl_reset_reviewflag','file')==2,tl_reset_reviewflag(gcbh);end  DeleteFcn=if exist('delete_tlblock','file')==2,delete_tlblock(gcbh);end  NameChangeFcn=if exist('rename_tlblock','file')==2,rename_tlblock(gcbh);end  OpenFcn=if exist('tl_open_blockdlg','file')==2,tl_open_blockdlg(gcbh);else,open_system(gcbh,'parameter');end
      mask Help: eval(['if exist(''tl_online_help'',''file'') == 2, tl_online_help(''Topic'',''TL_Product''),else, web([''jar:file:///'',matlabroot,''/help/toolbox/simulink/help.jar!/slref/' lower(get_param(gcbh,'Blocktype')) '.html''], ''-helpbrowser''),end'])
      mask Display: plot([-0.05, 1.05, NaN, -0.05, 1.05],[.01, .01, NaN, .99, .99])
  Relational Operator : RelationalOperator  Operator===  OutDataTypeStr=boolean  mask(TL_RelationalOperator){data={'date',735951.66799305554}}
      settings: DeleteFcn=if exist('delete_tlblock','file')==2,delete_tlblock(gcbh);end  NameChangeFcn=if exist('rename_tlblock','file')==2,rename_tlblock(gcbh);end  OpenFcn=if exist('tl_open_blockdlg','file')==2,tl_open_blockdlg(gcbh);else,open_system(gcbh,'parameter');end
      mask Help: eval(['if exist(''tl_online_help'',''file'') == 2, tl_online_help(''Topic'',''TL_RelationalOperator''),else, web([''jar:file:///'',matlabroot,''/help/toolbox/simulink/help.jar!/slref/' lower(get_param(gcbh,'Blocktype')) '.html''], ''-helpbrowser''),end'])
      mask Display: plot([-0.05, 1.05, NaN, -0.05, 1.05],[.01, .01, NaN, .99, .99])
  Switch : Switch  Criteria=u2 ~= 0  mask(TL_Switch){data={'output',{'name','u8FilteredPowerDegFactor','type','UInt8'},'date',735951.66799276625}}
      settings: CopyFcn=if exist('tl_reset_reviewflag','file')==2,tl_reset_reviewflag(gcbh);end  DeleteFcn=if exist('delete_tlblock','file')==2,delete_tlblock(gcbh);end  NameChangeFcn=if exist('rename_tlblock','file')==2,rename_tlblock(gcbh);end  OpenFcn=if exist('tl_open_blockdlg','file')==2,tl_open_blockdlg(gcbh);else,open_system(gcbh,'parameter');end
      mask Help: eval(['if exist(''tl_online_help'',''file'') == 2, tl_online_help(''Topic'',''TL_Switch''),else, web([''jar:file:///'',matlabroot,''/help/toolbox/simulink/help.jar!/slref/' lower(get_param(gcbh,'Blocktype')) '.html''], ''-helpbrowser''),end'])
      mask Display: plot([-0.05, 1.05, NaN, -0.05, 1.05],[.01, .01, NaN, .99, .99])
  Temperature Weighted : Subsystem  TreatAsAtomicUnit=on
  s32_CorrectedOrderValue : Outport
  wires:
  u8_OrderType/1 -> Relational Operator/2
  PWM order type key value/1 -> Relational Operator/1
  Relational Operator/1 -> Switch/2
  KU8_NO_POWER_ADAPT/1 -> Switch/1
  u8_PowerDegradationFactor/1 -> Switch/3
  s8_StepOrderValue/1 -> Temperature Weighted/1(s8_StepOrderValue), Product2/2
  e_TemperatureCompensationType/1 -> Temperature Weighted/3(e_TemperatureCompensationType)
  u16_Temperature/1 -> Temperature Weighted/2(u16_Temperature)
  b_IsWeightedStep/1 -> If/1
  If/1 -> Temperature Weighted/Action
  If/2 -> No Temperature Adaptation/Action
  No Temperature Adaptation/1(Out1) -> Merge/1
  Temperature Weighted/1(Out1) -> Merge/2
  Product1/1 -> s32_CorrectedOrderValue/1
  Switch/1 -> Product2/1
  Merge/1 -> Product1/2
  Product2/1 -> Product1/1
